simulink model "diabetes_2slxComputer"  (R2023b)
settings: Solver=FixedStepAuto  StartTime=0.0  StopTime=100  RelTol=1e-3  EnableMultiTasking=on
StopFcn:
  | plot_results
undefined symbols (not defined in the file or in its folder): Standard_Devices, UDP_Protocol
libraries: sldrtlib x2, simulink x1, realtime_pacer_lib x1
settings Model: Creator=tsladeche  LastModifiedBy=ryanmccord
settings SolverCC: AlgebraicLoopSolver=TrustRegion  PositivePriorityOrder=on
settings DataIOCC: LimitDataPoints=on  SaveFormat=Array  SignalLoggingSaveFormat=ModelDataLogs  ReturnWorkspaceOutputs=off
settings OptimizationCC: DefaultParameterBehavior=Inlined  EnhancedBackFolding=on  PassReuseOutputArgsThreshold=0  ExpressionDepthLimit=2147483647  MaxStackSize=64  OptimizeBlockOrder=speed  DifferentSizesBufferReuse=on  OptimizationCustomize=off
settings DebuggingCC: UnderspecifiedInitializationDetection=Classic  MergeDetectMultiDrivingBlocksExec=none  SolverPrmCheckMsg=warning  ParameterTunabilityLossMsg=error  FcnCallInpInsideContextMsg=warning  UnconnectedInputMsg=warning  UnconnectedOutputMsg=warning  UnconnectedLineMsg=warning  StateNameClashWarn=warning  SFUnexpectedBacktrackingDiag=warning  SFNoUnconditionalDefaultTransitionDiag=warning  SFExecutionAtInitializationDiag=none  ArithmeticOperatorsInVariantConditions=warning
settings HardwareCC: ProdBitPerLong=64  ProdHWDeviceType=Intel->x86-64 (Linux 64)
settings ModelReferenceCC: PropagateSignalLabelsOutOfModel=off
settings SFSimCC: SimUseLocalCustomCode=off  CustomCodeUndefinedFunction=UseInterfaceOnly
settings RTWCC: Description=Simulink Desktop Real-Time  SystemTargetFile=sldrt.tlc  TemplateMakefile=sldrt.tmf  RTWUseLocalCustomCode=off  Toolchain=GNU GCC Embedded Linux  BuildConfiguration=Faster Runs  RTWCompilerOptimization=on
settings CodeAppCC: ForceParamTrailComments=on  MaxIdLength=95  OperatorAnnotations=on
settings SimulinkDesktopRealTimeCC: TargetLibSuffix=_sldrt.a  TargetPreCompLibLocation=/Applications/MATLAB_R2023b.app/toolbox/sldrt/lib/maci64  TargetLangStandard=C89/C90 (ANSI)
settings ConfigComp: CovMetricSettings=dw  CovSaveCumulativeToWorkspaceVar=on  CovSaveSingleToWorkspaceVar=on  CovExternalEMLEnable=off

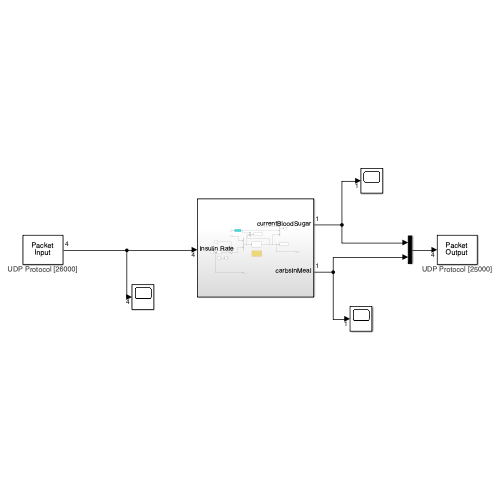
[thumbnail: Simulink's stored preview of the top-level diagram]
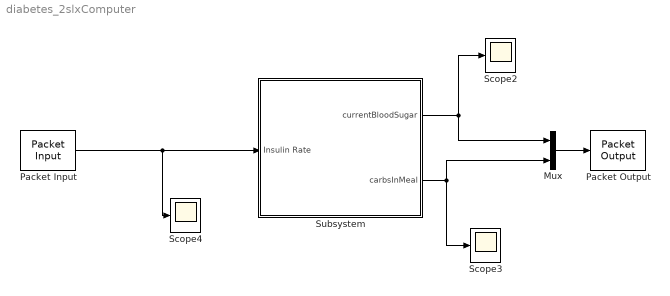
== system diabetes_2slxComputer ==
  Mux : Mux  Inputs=2
  Packet Input : sldrtlib/Packet Input  SampleTime=0.1  MaxMissedTicks=10  ShowMissedTicks=off  YieldWhenWaiting=off  DrvName=Standard_Devices/UDP_Protocol  DrvAddress=26000  DrvOptions=[0 0 114 97 115 112 98 101 114 114 121 112 105 46 108 111 99 97 108 0 0 0 0 0 0 0 0 0 0 0 0 0 0 0 0 0 0 0 0 0 0 0 0 0 0 0 0 0 0 0 0 0 0 0 0 0 0 0 0 0 0 0 0 0 0 0 0 0 0 0 0 0 0 0 0 0 0 0 0 0 0 0 0 0 0 0 0 0 0 0 0 0 0 0 0 0 0 0 0 0 0 0 0 0 0 0 0 0 0 0 0 0 0 0 0 0 0 0 0 0 0 0 0 0 0 0 0 0 0 0 0 0 0 0 0 0 0 0 0 0 0 0 0 0 0 0 0 0 0 0 0 0 0 0 0 0 0 0 0 0 0 0 0 0 0 0 0 0 0 0 0 0 0 0 0 0 0 0 0 0 0 0 0 0 0 0 0 0 0 0 0 0 0 0 0 0 0 0 0 0 0 0 0 0 0 0 0 0 0 0 0 0 0 0 0 0 0 0 0 0 0 0 0 0 0 0 0 0 0 0 0 0 0 0 0 0 0 0 0 0 0 0 0 0 0 0 0 0 0 0 0 0 0 0 0 0]  PacketSize=32  DataTypes='4*double'  ShowReady=off  ShowError=off  PacketID=1  ByteOrder=1  ShowTimestamp=off
      settings: AttributesFormatString=UDP Protocol [26000]
  Packet Output : sldrtlib/Packet Output  SampleTime=0.1  MaxMissedTicks=10  ShowMissedTicks=off  YieldWhenWaiting=off  DrvName=Standard_Devices/UDP_Protocol  DrvAddress=25000  DrvOptions=[0 0 114 97 115 112 98 101 114 114 121 112 105 46 108 111 99 97 108 0 0 0 0 0 0 0 0 0 0 0 0 0 0 0 0 0 0 0 0 0 0 0 0 0 0 0 0 0 0 0 0 0 0 0 0 0 0 0 0 0 0 0 0 0 0 0 0 0 0 0 0 0 0 0 0 0 0 0 0 0 0 0 0 0 0 0 0 0 0 0 0 0 0 0 0 0 0 0 0 0 0 0 0 0 0 0 0 0 0 0 0 0 0 0 0 0 0 0 0 0 0 0 0 0 0 0 0 0 0 0 0 0 0 0 0 0 0 0 0 0 0 0 0 0 0 0 0 0 0 0 0 0 0 0 0 0 0 0 0 0 0 0 0 0 0 0 0 0 0 0 0 0 0 0 0 0 0 0 0 0 0 0 0 0 0 0 0 0 0 0 0 0 0 0 0 0 0 0 0 0 0 0 0 0 0 0 0 0 0 0 0 0 0 0 0 0 0 0 0 0 0 0 0 0 0 0 0 0 0 0 0 0 0 0 0 0 0 0 0 0 0 0 0 0 0 0 0 0 0 0 0 0 0 0 0 0]  PacketSize=32  DataTypes='4*double'  ShowReady=off  ShowError=off  PacketID=1  ByteOrder=1  InitialValue=[]  FinalValue=[]
      settings: AttributesFormatString=UDP Protocol [25000]
  Scope2 : Scope
  Scope3 : Scope
  Scope4 : Scope
  Subsystem : Subsystem
  wires:
  Subsystem/2(carbsInMeal) -> Mux/2, Scope3/1
  Subsystem/1(currentBloodSugar) -> Mux/1, Scope2/1
  Mux/1 -> Packet Output/1
  Packet Input/1 -> Scope4/1, Subsystem/1(Insulin Rate)

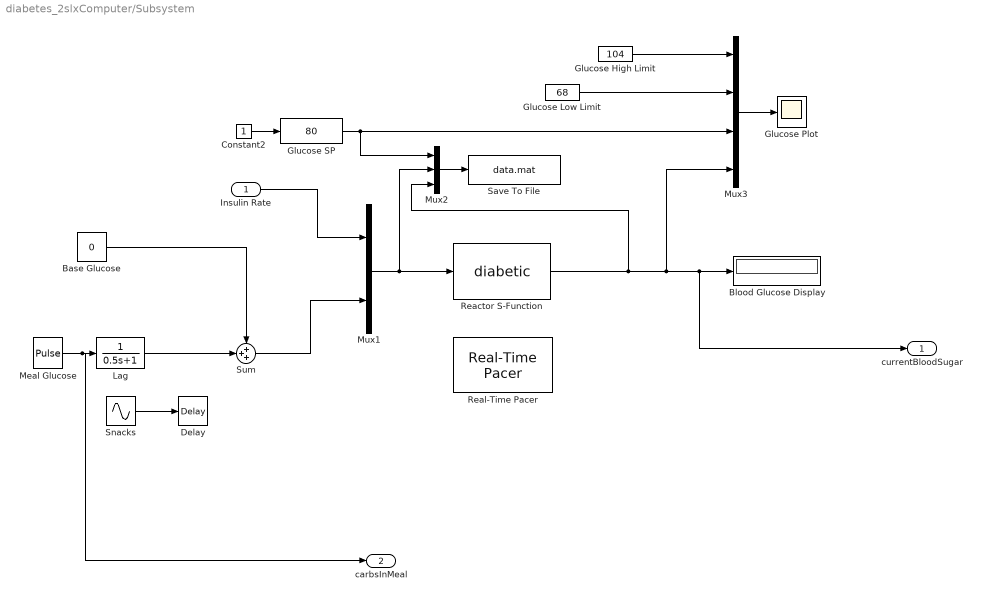
== system diabetes_2slxComputer/Subsystem ==
  Insulin Rate : Inport
  Base Glucose : Constant  Value=0
  Blood Glucose Display : Display
  Constant2 : Constant
  Delay : TransportDelay  DelayTime=8
  Glucose High Limit : Constant  Value=104
  Glucose Low Limit : Constant  Value=68
  Glucose Plot : Scope
  Glucose SP : simulink/Math Operations/Slider Gain  gain=80  low=50  high=120
  Lag : TransferFcn  Denominator=[0.5 1]
  Meal Glucose : DiscretePulseGenerator  PulseType=Time based  Amplitude=60  Period=30  PulseWidth=20  PhaseDelay=7
  Mux1 : Mux  Inputs=2
  Mux2 : Mux  Inputs=3
  Mux3 : Mux
  Reactor S-Function : S-Function  FunctionName=diabetic  SFunctionDeploymentMode=off  EnableBusSupport=off
  Real-Time Pacer : realtime_pacer_lib/Real-Time Pacer  simTimePerRealTime=1
      settings: SourceProductName=Real-Time Pacer
  Save To File : ToFile  Filename=data.mat  MatrixName=diabetic  SampleTime=0.05
  Snacks : Sin  Amplitude=50  SampleTime=0
  Sum : Sum  Inputs=+++
  currentBloodSugar : Outport
  carbsInMeal : Outport  Port=2
  wires:
  Snacks/1 -> Delay/1
  Sum/1 -> Mux1/2
  Reactor S-Function/1 -> Mux3/4, currentBloodSugar/1, Blood Glucose Display/1, Mux2/3
  Meal Glucose/1 -> carbsInMeal/1, Lag/1
  Mux1/1 -> Mux2/2, Reactor S-Function/1
  Constant2/1 -> Glucose SP/1
  Glucose SP/1 -> Mux3/3, Mux2/1
  Base Glucose/1 -> Sum/1
  Insulin Rate/1 -> Mux1/1
  Glucose Low Limit/1 -> Mux3/2
  Lag/1 -> Sum/2
  Mux3/1 -> Glucose Plot/1
  Mux2/1 -> Save To File/1
  Glucose High Limit/1 -> Mux3/1
